simulink model "PWM_PPM"  (R2024a)
settings: Solver=VariableStepAuto  StartTime=0.0  StopTime=10.0  RelTol=1e-3
libraries: simulink x2, spsBistableLib x1, spsMonostableLib x1
settings Model: Creator=adity  LastModifiedBy=adity

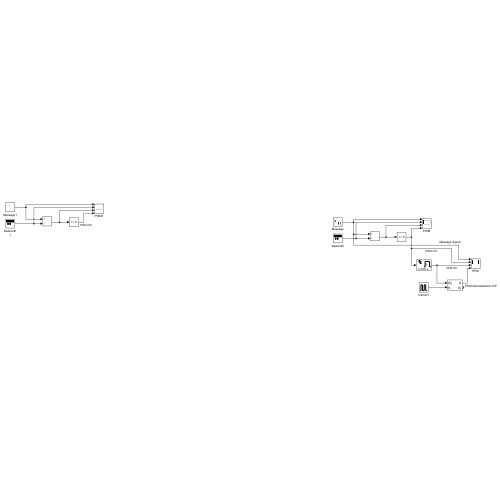
[thumbnail: Simulink's stored preview of the top-level diagram]
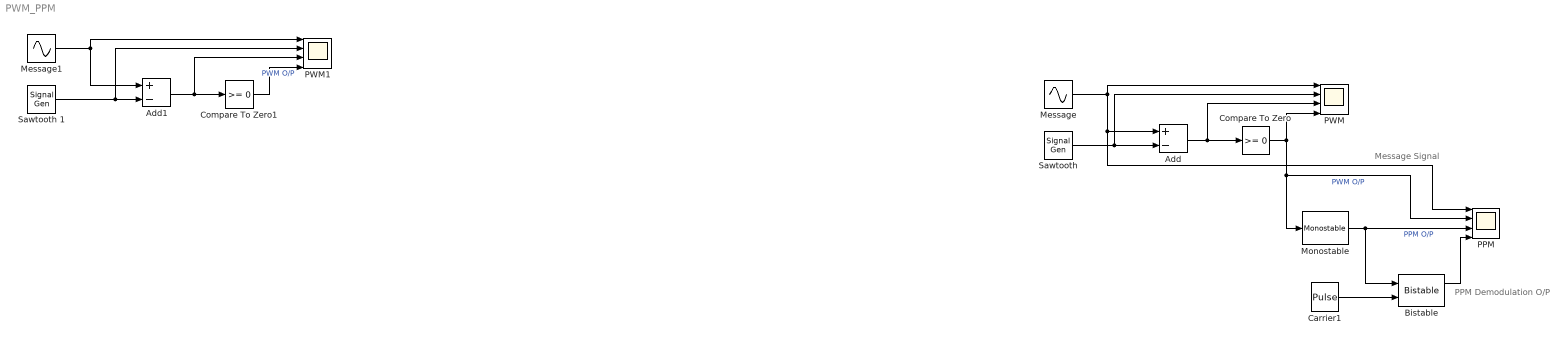
== system PWM_PPM ==
  note: PPM Demodulation O/P
  note: Message Signal
  Add : Sum  Inputs=+-
  Add1 : Sum  Inputs=+-
  Bistable : spsBistableLib/Bistable  Qpriority=Set  ic=0  Ts=0
      settings: LibrarySourceBlock=sps_lib/Control/Bistable
  Carrier1 : DiscretePulseGenerator  PulseType=Time based  Period=0.02  PulseWidth=50
  Compare To Zero : simulink/Logic and Bit Operations/Compare To Zero  relop=>=  OutDataTypeStr=boolean
  Compare To Zero1 : simulink/Logic and Bit Operations/Compare To Zero  relop=>=  OutDataTypeStr=boolean
  Message : Sin  Frequency=2*pi*1  SampleTime=1/1000
  Message1 : Sin  Frequency=2*pi*1  SampleTime=1/1000
  Monostable : spsMonostableLib/Monostable  EdgeDetect=Falling  PulseDuration=0.015  ic=0  Ts=0
      settings: LibrarySourceBlock=sps_lib/Control/Monostable
  PPM : Scope  NumInputPorts=4
  PWM : Scope  NumInputPorts=4
  PWM1 : Scope  NumInputPorts=4
  "Sawtooth " : SignalGenerator  WaveForm=sawtooth  Frequency=10
  Sawtooth 1 : SignalGenerator  WaveForm=sawtooth  Frequency=10
  wires:
  Message/1 -> PPM/1, Add/1, PWM/1
  Compare To Zero/1 -> PWM/4, PPM/2, Monostable/1  "PWM O/P"
  Monostable/1 -> PPM/3, Bistable/1  "PPM O/P"
  "Sawtooth "/1 -> PWM/2, Add/2
  Add/1 -> Compare To Zero/1, PWM/3
  Carrier1/1 -> Bistable/2
  Bistable/1 -> PPM/4
  Compare To Zero1/1 -> PWM1/4  "PWM O/P"
  Message1/1 -> Add1/1, PWM1/1
  Add1/1 -> PWM1/3, Compare To Zero1/1
  Sawtooth 1/1 -> PWM1/2, Add1/2
